simulink model "eTractor_KRAKER_etrailer_v2_2"  (R2023a)
settings: Solver=VariableStepAuto  StartTime=0.0  StopTime=tmax  FixedStep=dt  RelTol=1e-4  EnableMultiTasking=on
PreLoadFcn:
  | init_vehicle
  | init_ETruck
  | init_SIMULATION_runfile
StartFcn:
  | tic
StopFcn:
  | toc
  | sim_stop_function
values from neighbouring files (symbols this model uses):
  Arms = [100 200 300 400 500 600]    [init_BURGERS.m]    (also in init_KRAKER.m)
  brake_input = [0   tmax ... (first row only)    [init_vehicle.m]    (also in run_Circle.m = [0  tmax; run_Coastdown.m = [0  2  tmax; run_DoubleLaneChangeDriver.m = [0   2  tmax; run_MaxAcc.m = [0  2  tmax)
  chassis_length = 13.82    [init_BURGERS.m]    (also in init_KRAKER.m = 10.36)
  energyCapacity = 116.89    [init_BURGERS.m]    (also in init_KRAKER.m)
  etrailer_ON = 1    [init_SIMULATION_runfile.m]
  ETruck_energyCapacity = 650    [init_ETruck.m]
  ETruck_G_motor = 17.5    [init_ETruck.m]
  ETruck_initialSOC = 0.95    [init_ETruck.m]
  ETruck_MaxTrqOut = 2250    [init_ETruck.m]
  ETruck_Std_Regen_Trq = 300    [init_ETruck.m]
  ETruck_Voc = 750    [init_ETruck.m]
  front_overhang = 1.620    (= 1.62)    [init_BURGERS.m]    (also in init_KRAKER.m = 1.305)
  G_diff = 1    [init_BURGERS.m]    (also in init_KRAKER.m = 6)
  initialSOC = 0.95    [init_BURGERS.m]    (also in init_KRAKER.m = 0.65)
  InputSwitch = 2    [init_SIMULATION_runfile.m]
  inverter_thermal_res = 0.017    [init_BURGERS.m]    (also in init_KRAKER.m)
  L_0f = 3.8    [init_vehicle.m]
  LD = 1    [init_vehicle.m]
  mass = mass_trailer    (= 11000)    [init_BURGERS.m]    (also in init_KRAKER.m = 7350; run_Statics_MF_MAT.m = (Fz_front_axle1+Fz_rear_axle1+       Fz_trailer1_axle1+Fz_tr; run_Statics_MF_TNO.m = (Fz_front_axle1+Fz_rear_axle1+       Fz_trailer1_axle1+Fz_tr)
  massload = 23000    [init_SIMULATION_runfile.m]
  MaxTrqOut = 525    [init_BURGERS.m]    (also in init_KRAKER.m = 950)
  outside_temp = 25    [init_BURGERS.m]    (also in init_KRAKER.m)
  pose_t0 = [0 0 0 0]    [init_vehicle.m]    (also in run_Circle.m; run_Coastdown.m; run_DoubleLaneChangeDriver.m; run_MaxAcc.m)
  Power_dissipation = [261 384 513 642; 552 783 1020 1260; 894 1233 1584 1956; 1300 1750 2200 2740; 1740 2300 2900 3550; 2250 2900 3650 4500]    [init_BURGERS.m]    (also in init_KRAKER.m)
  sp_t = 0.01    [init_vehicle.m]
  Std_Regen_Trq = 300    [init_BURGERS.m]    (also in init_KRAKER.m)
  steer_input = [0  tmax ... (first row only)    [init_vehicle.m]    (also in run_Circle.m = [0  2   10     13       tmax; run_Coastdown.m = [0 tmax; run_DoubleLaneChangeDriver.m = [0 tmax; run_MaxAcc.m = [0 tmax)
  steer_ratio = 20    [init_vehicle.m]
  steer_sens = 1    [init_vehicle.m]
  throttle_input = [0         tmax ... (first row only)    [init_vehicle.m]    (also in run_Circle.m; run_Coastdown.m = [0        10         10.0001 tmax; run_DoubleLaneChangeDriver.m = [0        tmax; run_MaxAcc.m = [0        tmax)
  tire_param_drive = simscape.multibody.tirread('DRIVE_315_70R22.5_9b_MF62.tir')    [init_vehicle.m]
  tire_param_steer = simscape.multibody.tirread('STEER_315_70R22.5_9b_MF62.tir')    [init_vehicle.m]
  tire_param_trailer = simscape.multibody.tirread('TRAILER_385_65R22.5_9b0_MF62.tir')    [init_vehicle.m]
  tire_width = 0.318    [init_vehicle.m]
  trailer_ID = 1    [init_SIMULATION_runfile.m]
  v_0 = 1    [init_vehicle.m]
  Vdc = [200 400 600 800]    [init_BURGERS.m]    (also in init_KRAKER.m)
  Voc = 675    [init_BURGERS.m]    (also in init_KRAKER.m)
  Vx = 0    [init_vehicle.m]    (also in run_Circle.m = Vx_kmh/3.6; run_Coastdown.m = Vx_kmh/3.6; run_DoubleLaneChangeDriver.m = Vx_kmh/3.6; run_MaxAcc.m)
  Vx_input = [0  tmax ... (first row only)    [init_vehicle.m]    (also in run_Circle.m; run_Coastdown.m = [0 tmax; run_DoubleLaneChangeDriver.m = [0 tmax; run_MaxAcc.m = [0 tmax)
  wheelbase = 8.115    [init_BURGERS.m]    (also in init_KRAKER.m = 5.584)
undefined symbols (not defined in the file or in its folder): end_val, final_x, final_y, Floor, steer_path, X, Y, Z
libraries: sm_lib x367, nesl_utility x289, fl_lib x29, sdl_lib x4, batteryecm_lib x2, ee_lib x2, BatteryEstimators x2, robotalgslib x1, simulink_extras x1, CommercialVehicleLibrary2G x1
(part 9 of 14)

== system eTractor_KRAKER_etrailer_v2_2/Tractor_semitrailer /e-Tractor/World ==
  note: Road Vizualisation
  " pos_initial" : sm_lib/Frames and Transforms/Rigid Transform  TranslationMethod=Cartesian  TranslationStandardOffset=0  TranslationStandardOffsetUnits=m  TranslationStandardAxis=+Z  TranslationCartesianOffset=[Xt0 Yt0 0]  TranslationCartesianOffsetUnits=m  TranslationROffset=0  TranslationROffsetUnits=m  TranslationZOffset=0  TranslationZOffsetUnits=m  TranslationThetaOffset=0  TranslationThetaOffsetUnits=deg  RotationMethod=StandardAxis  RotationAngleUnits=deg  RotationStandardAxis=+Z  RotationAngle=Psit0  RotationArbitraryAxis=[0 0 1]  FollAlignAxisA=+X  BaseAlignAxisA=+Y  FollAlignAxisB=+Y  BaseAlignAxisB=+Z  RotationSequenceAxes=FollowerAxes  RotationSequence=XYX  RotationSequenceAngles=[0 0 0]  RotationSequenceAnglesUnits=deg  RotationMatrix=[1 0 0; 0 1 0; 0 0 1]  Quaternion=[1 0 0 0]
  6-DOF Joint : sm_lib/Joints/6-DOF Joint  JointMode=Normal  SenseConstraintForce=off  SenseConstraintForceX=off  SenseConstraintForceY=off  SenseConstraintForceZ=off  SenseConstraintTorque=off  SenseConstraintTorqueX=off  SenseConstraintTorqueY=off  SenseConstraintTorqueZ=off  SenseTotalForce=off  SenseTotalForceX=off  SenseTotalForceY=off  SenseTotalForceZ=off  SenseTotalTorque=off  SenseTotalTorqueX=off  SenseTotalTorqueY=off  SenseTotalTorqueZ=off  CompositeWrenchDir=BaseOnFollower  CompositeWrenchFrame=BaseFrame  PxEquilibriumPosition=0  PxEquilibriumPositionUnits=m  PxSpringStiffness=0  PxSpringStiffnessUnits=N/m  PxDampingCoefficient=0  PxDampingCoefficientUnits=N/(m/s)  PxTorqueActuationMode=NoTorque  PxMotionActuationMode=ComputedMotion  PxSensePosition=on  PxSenseVelocity=off  PxSenseAcceleration=off  PxSenseTorqueForce=off  PxSenseLowerLimitTorqueForce=off  PxSenseUpperLimitTorqueForce=off  PxLowerLimitSpecify=off  PxLowerLimitBound=-1  PxLowerLimitBoundUnits=m  PxLowerLimitStiffness=1e6  PxLowerLimitStiffnessUnits=N/m  PxLowerLimitDamping=1e3  PxLowerLimitDampingUnits=N/(m/s)  PxLowerLimitTransitionRegionWidth=1e-4  PxLowerLimitTransitionRegionWidthUnits=m  PxUpperLimitSpecify=off  PxUpperLimitBound=1  PxUpperLimitBoundUnits=m  PxUpperLimitStiffness=1e6  PxUpperLimitStiffnessUnits=N/m  PxUpperLimitDamping=1e3  PxUpperLimitDampingUnits=N/(m/s)  PxUpperLimitTransitionRegionWidth=1e-4  PxUpperLimitTransitionRegionWidthUnits=m  PxPositionTargetSpecify=off  PxPositionTargetPriority=High  PxPositionTargetValue=0  PxPositionTargetValueUnits=m  PxVelocityTargetSpecify=off  PxVelocityTargetPriority=High  PxVelocityTargetValue=Vx  PxVelocityTargetValueUnits=m/s  PyEquilibriumPosition=0  PyEquilibriumPositionUnits=m  PySpringStiffness=0  PySpringStiffnessUnits=N/m  PyDampingCoefficient=0  PyDampingCoefficientUnits=N/(m/s)  PyTorqueActuationMode=NoTorque  PyMotionActuationMode=ComputedMotion  PySensePosition=on  PySenseVelocity=off  PySenseAcceleration=off  PySenseTorqueForce=off  PySenseLowerLimitTorqueForce=off  PySenseUpperLimitTorqueForce=off  PyLowerLimitSpecify=off  PyLowerLimitBound=-1  PyLowerLimitBoundUnits=m  PyLowerLimitStiffness=1e6  PyLowerLimitStiffnessUnits=N/m  PyLowerLimitDamping=1e3  PyLowerLimitDampingUnits=N/(m/s)  PyLowerLimitTransitionRegionWidth=1e-4  PyLowerLimitTransitionRegionWidthUnits=m  PyUpperLimitSpecify=off  PyUpperLimitBound=1  PyUpperLimitBoundUnits=m  PyUpperLimitStiffness=1e6  PyUpperLimitStiffnessUnits=N/m  PyUpperLimitDamping=1e3  PyUpperLimitDampingUnits=N/(m/s)  PyUpperLimitTransitionRegionWidth=1e-4  PyUpperLimitTransitionRegionWidthUnits=m  PyPositionTargetSpecify=off  PyPositionTargetPriority=High  PyPositionTargetValue=0  PyPositionTargetValueUnits=m  PyVelocityTargetSpecify=off  PyVelocityTargetPriority=High  PyVelocityTargetValue=0  PyVelocityTargetValueUnits=m/s  PzEquilibriumPosition=0  PzEquilibriumPositionUnits=m  PzSpringStiffness=0  PzSpringStiffnessUnits=N/m  PzDampingCoefficient=0  PzDampingCoefficientUnits=N/(m/s)  PzTorqueActuationMode=NoTorque  PzMotionActuationMode=ComputedMotion  PzSensePosition=on  PzSenseVelocity=off  PzSenseAcceleration=off  PzSenseTorqueForce=off  PzSenseLowerLimitTorqueForce=off  PzSenseUpperLimitTorqueForce=off  PzLowerLimitSpecify=off  PzLowerLimitBound=-1  PzLowerLimitBoundUnits=m  PzLowerLimitStiffness=1e6  PzLowerLimitStiffnessUnits=N/m  PzLowerLimitDamping=1e3  PzLowerLimitDampingUnits=N/(m/s)  PzLowerLimitTransitionRegionWidth=1e-4  PzLowerLimitTransitionRegionWidthUnits=m  PzUpperLimitSpecify=off  PzUpperLimitBound=1  PzUpperLimitBoundUnits=m  PzUpperLimitStiffness=1e6  PzUpperLimitStiffnessUnits=N/m  PzUpperLimitDamping=1e3  PzUpperLimitDampingUnits=N/(m/s)  PzUpperLimitTransitionRegionWidth=1e-4  PzUpperLimitTransitionRegionWidthUnits=m  PzPositionTargetSpecify=off  PzPositionTargetPriority=High  PzPositionTargetValue=0  PzPositionTargetValueUnits=m  PzVelocityTargetSpecify=off  PzVelocityTargetPriority=High  PzVelocityTargetValue=0  PzVelocityTargetValueUnits=m/s  SphEqPosRotationMethod=None  SphEqPosRotationAngleUnits=deg  SphEqPosRotationStandardAxis=+Z  SphEqPosRotationAngle=0.0  SphEqPosRotationArbitraryAxis=[0 0 1]  SphEqPosFollAlignAxisA=+X  SphEqPosBaseAlignAxisA=+Y  SphEqPosFollAlignAxisB=+Y  SphEqPosBaseAlignAxisB=+Z  SphEqPosRotationSequenceAxes=FollowerAxes  SphEqPosRotationSequence=XYX  SphEqPosRotationSequenceAngles=[0 0 0]  SphEqPosRotationSequenceAnglesUnits=deg  SphEqPosRotationMatrix=[1 0 0; 0 1 0; 0 0 1]  SphEqPosQuaternion=[1 0 0 0]  SphSpringStiffness=0  SphSpringStiffnessUnits=N*m/deg  SphDampingCoefficient=0  SphDampingCoefficientUnits=N*m/(deg/s)  SphActuateTorqueX=off  SphActuateTorqueY=off  SphActuateTorqueZ=off  SphActuateTorque=off  SphTorqueActuationMode=NoTorque  SphMotionActuationMode=ComputedMotion  SphActuationFrame=BaseFrame  SphSensePosition=off  SphSenseVelocityX=off  SphSenseVelocityY=off  SphSenseVelocityZ=off  SphSenseVelocity=off  SphSenseAccelerationX=off  SphSenseAccelerationY=off  SphSenseAccelerationZ=off  SphSenseAcceleration=off  SphSenseTorqueX=off  SphSenseTorqueY=off  SphSenseTorqueZ=off  SphSenseTorqueForce=off  SphSenseLowerLimitTorqueMag=off  SphSenseUpperLimitTorqueMag=off  SphSensingFrame=BaseFrame  SphLowerLimitSpecify=off  SphLowerLimitBound=15  SphLowerLimitBoundUnits=deg  SphLowerLimitStiffness=1e4  SphLowerLimitStiffnessUnits=N*m/deg  SphLowerLimitDamping=10  SphLowerLimitDampingUnits=N*m/(deg/s)  SphLowerLimitTransitionRegionWidth=0.1  SphLowerLimitTransitionRegionWidthUnits=deg  SphUpperLimitSpecify=off  SphUpperLimitBound=45  SphUpperLimitBoundUnits=deg  SphUpperLimitStiffness=1e4  SphUpperLimitStiffnessUnits=N*m/deg  SphUpperLimitDamping=10  SphUpperLimitDampingUnits=N*m/(deg/s)  SphUpperLimitTransitionRegionWidth=0.1  SphUpperLimitTransitionRegionWidthUnits=deg  SphPositionTargetRotationMethod=None  SphPositionTargetRotationAngleUnits=deg  SphPositionTargetRotationStandardAxis=+Z  SphPositionTargetRotationAngle=0.0  SphPositionTargetRotationArbitraryAxis=[0 0 1]  SphPositionTargetFollAlignAxisA=+X  SphPositionTargetBaseAlignAxisA=+Y  SphPositionTargetFollAlignAxisB=+Y  SphPositionTargetBaseAlignAxisB=+Z  SphPositionTargetRotationSequenceAxes=FollowerAxes  SphPositionTargetRotationSequence=XYX  SphPositionTargetRotationSequenceAngles=[0 0 0]  SphPositionTargetRotationSequenceAnglesUnits=deg  SphPositionTargetRotationMatrix=[1 0 0; 0 1 0; 0 0 1]  SphPositionTargetQuaternion=[1 0 0 0]  SphPositionTargetSpecify=off  SphPositionTargetPriority=High  SphVelocityTargetValue=[0 0 0]  SphVelocityTargetValueUnits=deg/s  SphVelocityTargetSpecify=off  SphVelocityTargetPriority=High  SphVelocityTargetInFollowerFrame=on
  Bus Creator1 : BusCreator  Inputs=6
  Constant1 : Constant  Commented=on  Value=5000
  Floor : sm_lib/Body Elements/Brick Solid  GraphicAmbientColor=[0.15 0.15 0.15 1.0]  BasedOnType=Density  BrickDimensions=[Floor.l , Floor.w , Floor.h]  BrickDimensionsUnits=m  CenterOfMass=[0 0 0]  CenterOfMassUnits=m  GraphicDiffuseColor=[0.6 0.6 0.6]  Density=1000  DensityUnits=kg/(m^3)  DoExposeReferenceFrame=on  GraphicEmissiveColor=[0.0 0.0 0.0 1.0]  ExportEntireGeometry=off  SerializedFrames=<Frames/>  MarkerShape=Sphere  MarkerSize=10  GraphicType=FromGeometry  InertiaType=CalculateFromGeometry  Mass=1  MassUnits=kg  MomentsOfInertia=[1 1 1]  MomentsOfInertiaUnits=kg*m^2  GraphicOpacity=1.0  ProductsOfInertia=[0 0 0]  ProductsOfInertiaUnits=kg*m^2  GraphicShininess=75  GraphicSpecularColor=[0.5 0.5 0.5 1.0]  GraphicVisPropType=AdvancedVisualProperties
  Grid XLines : sm_lib/Body Elements/Extruded Solid  GraphicAmbientColor=[0.15 0.15 0.15 1.0]  BasedOnType=Density  CenterOfMass=[0 0 0]  CenterOfMassUnits=m  GraphicDiffuseColor=Grid.clr  ExportConvexHullGeometry=off  ExtrusionCrossSection=Grid.extr_data  ExtrusionCrossSectionUnits=m  Density=1000  DensityUnits=kg/m^3  DoExposeReferenceFrame=on  GraphicEmissiveColor=[0.0 0.0 0.0 1.0]  ExportEntireGeometry=off  ExtrusionLength=Floor.h*1.005  ExtrusionLengthUnits=m  ExtrusionType=General  SerializedFrames=<Frames/>  MarkerShape=Sphere  MarkerSize=10  GraphicType=FromGeometry  InertiaType=PointMass  Mass=1  MassUnits=kg  MomentsOfInertia=[1 1 1]  MomentsOfInertiaUnits=kg*m^2  PolygonNumSides=3  GraphicOpacity=1.0  PolygonOuterRadius=1  PolygonOuterRadiusUnits=m  ProductsOfInertia=[1 1 1]  ProductsOfInertiaUnits=kg*m^2  GraphicShininess=75  GraphicSpecularColor=[0.5 0.5 0.5 1.0]  GraphicVisPropType=SimpleVisualProperties
  Grid YLines : sm_lib/Body Elements/Extruded Solid  GraphicAmbientColor=[0.15 0.15 0.15 1.0]  BasedOnType=Density  CenterOfMass=[0 0 0]  CenterOfMassUnits=m  GraphicDiffuseColor=Grid.clr  ExportConvexHullGeometry=off  ExtrusionCrossSection=Grid.extr_data  ExtrusionCrossSectionUnits=m  Density=1000  DensityUnits=kg/m^3  DoExposeReferenceFrame=on  GraphicEmissiveColor=[0.0 0.0 0.0 1.0]  ExportEntireGeometry=off  ExtrusionLength=Floor.h*1.005  ExtrusionLengthUnits=m  ExtrusionType=General  SerializedFrames=<Frames/>  MarkerShape=Sphere  MarkerSize=10  GraphicType=FromGeometry  InertiaType=PointMass  Mass=1  MassUnits=kg  MomentsOfInertia=[1 1 1]  MomentsOfInertiaUnits=kg*m^2  PolygonNumSides=3  GraphicOpacity=1.0  PolygonOuterRadius=1  PolygonOuterRadiusUnits=m  ProductsOfInertia=[1 1 1]  ProductsOfInertiaUnits=kg*m^2  GraphicShininess=75  GraphicSpecularColor=[0.5 0.5 0.5 1.0]  GraphicVisPropType=SimpleVisualProperties
  Infinite Plane : sm_lib/Curves and Surfaces/Infinite Plane  GraphicType=Rectangle  GraphicPlaneWidth=1  GraphicPlaneWidthUnits=m  GraphicPlaneHeight=1  GraphicPlaneHeightUnits=m  GraphicVisPropType=SimpleVisualProperties  GraphicDiffuseColor=[0.5 0.5 0.5]  GraphicOpacity=0.25  GraphicSpecularColor=[0.5 0.5 0.5 1.0]  GraphicAmbientColor=[0.15 0.15 0.15 1.0]  GraphicEmissiveColor=[0.0 0.0 0.0 1.0]  GraphicShininess=75
  Mechanism Configuration : sm_lib/Utilities/Mechanism Configuration  UniformGravity=Constant  GravityVector=[0 0 -9.81]  GravityVectorUnits=m/s^2  LinearizationDelta=0.001  JointModeTransitionNonlinearIterations=2
  PS-Simulink Converter : nesl_utility/PS-Simulink Converter  PhysicalDomain=network_engine_domain  SubClassName=ps_output  LeftPortType=input  RightPortType=output  PseudoPeriodic=off  Frequencies=[]  VectorFormat=1-D array  Unit=1  AffineConversion=off
  PS-Simulink Converter1 : nesl_utility/PS-Simulink Converter  PhysicalDomain=network_engine_domain  SubClassName=ps_output  LeftPortType=input  RightPortType=output  PseudoPeriodic=off  Frequencies=[]  VectorFormat=1-D array  Unit=m  AffineConversion=off
  PS-Simulink Converter2 : nesl_utility/PS-Simulink Converter  PhysicalDomain=network_engine_domain  SubClassName=ps_output  LeftPortType=input  RightPortType=output  PseudoPeriodic=off  Frequencies=[]  VectorFormat=1-D array  Unit=m  AffineConversion=off
  PS-Simulink Converter3 : nesl_utility/PS-Simulink Converter  PhysicalDomain=network_engine_domain  SubClassName=ps_output  LeftPortType=input  RightPortType=output  PseudoPeriodic=off  Frequencies=[]  VectorFormat=1-D array  Unit=m  AffineConversion=off
  "Road Grid Offset " : sm_lib/Frames and Transforms/Rigid Transform  TranslationMethod=Cartesian  TranslationStandardOffset=0  TranslationStandardOffsetUnits=m  TranslationStandardAxis=+Z  TranslationCartesianOffset=[0 0 -0.5*Floor.h]  TranslationCartesianOffsetUnits=m  TranslationROffset=0  TranslationROffsetUnits=m  TranslationZOffset=0  TranslationZOffsetUnits=m  TranslationThetaOffset=0  TranslationThetaOffsetUnits=deg  RotationMethod=None  RotationAngleUnits=deg  RotationStandardAxis=+Z  RotationAngle=45  RotationArbitraryAxis=[0 0 1]  FollAlignAxisA=+X  BaseAlignAxisA=+Y  FollAlignAxisB=+Y  BaseAlignAxisB=+Z  RotationSequenceAxes=FollowerAxes  RotationSequence=XYX  RotationSequenceAngles=[0 0 0]  RotationSequenceAnglesUnits=deg  RotationMatrix=[1 0 0; 0 1 0; 0 0 1]  Quaternion=[1 0 0 0]
  Simulink-PS Converter : nesl_utility/Simulink-PS Converter  Commented=on  PhysicalDomain=network_engine_domain  SubClassName=ps_input  LeftPortType=input  RightPortType=output  PseudoPeriodic=off  Frequencies=[]  NoiseDistribution=none  NoiseParameters=[]  Unit=N  AffineConversion=off  FilteringAndDerivatives=provide  SimscapeFilterOrder=1  InputFilterTimeConstant=0.001  UdotUserProvided=0
  Solver Configuration : nesl_utility/Solver Configuration  PhysicalDomain=network_engine_domain  SubClassName=solver  LeftPortType=input  RightPortType=generic  Tones=[]  Harmonics=[]  SimulateNoise=off  Profile=off  UseLocalSampling=off  EnableSwitchedLinearOptims=on  FrequencyDomain=off  UseCCode=off  RelTol=0.001  AbsTol=1e-06  MinStep=1e-09  ToWorkspace=off  RevertToSquareIcSolve=off  NumHomotopyIterations=100  PhasorMode=off  PhasorModeNumHarmonics=1  ConsistencySolver=NEWTON_FTOL  IndexReductionMethod=DerivativeReplacement  DoDC=off  ResidualTolerance=1e-09  ConsistencyTolSource=GLOBAL  ConsistencyAbsTol=0.001  ConsistencyRelTol=0.001  ConsistencyTolFactor=0.001  UseLocalSolver=off  LocalSolverChoice=NE_BACKWARD_EULER_ADVANCER  ResolveIndetEquations=on  FunctionEvalNumThread=1  LocalSolverSampleTime=0.001  DoFixedCost=off  MaxNonlinIter=3  MaxModeIter=2  ComputeImpulses=off  ImpulseIterations=2  LinearAlgebra=Sparse  LinearAlgebraNumThread=0  EquationFormulation=NE_TIME_EF  DelaysMemoryBudget=1024  AutomaticFiltering=on  FilteringTimeConstant=0.001  PartitionStorageMethod=AS_NEEDED  PartitionMemoryBudget=1024  PartitionMethod=ROBUST
  Step : Step  Commented=on  Time=10  After=25000  SampleTime=0
  Subsystem : Subsystem
      mask Display: disp('Yaw, Pitch & Roll');
  Transform Sensor : sm_lib/Frames and Transforms/Transform Sensor  MeasurementFrame=World  RotationSequence=XYX  SenseAngle=off  SenseAxis=off  SenseQ=off  SenseR=on  SenseRotationSequence=off  SenseOmegaX=off  SenseOmegaY=off  SenseOmegaZ=off  SenseQDot=off  SenseRDot=off  SenseRotationSequenceDot=off  SenseAlphaX=off  SenseAlphaY=off  SenseAlphaZ=off  SenseQDDot=off  SenseRDDot=off  SenseX=off  SenseY=off  SenseZ=off  SenseRad=off  SenseAzim=off  SenseDist=off  SenseInc=off  SenseXDot=off  SenseYDot=off  SenseZDot=off  SenseRadDot=off  SenseAzimDot=off  SenseDistDot=off  SenseIncDot=off  SenseXDDot=off  SenseYDDot=off  SenseZDDot=off  SenseRadDDot=off  SenseAzimDDot=off  SenseDistDDot=off  SenseIncDDot=off
  "Transform XLines " : sm_lib/Frames and Transforms/Rigid Transform  TranslationMethod=Cartesian  TranslationStandardOffset=0  TranslationStandardOffsetUnits=m  TranslationStandardAxis=+Z  TranslationCartesianOffset=[0 0 0]  TranslationCartesianOffsetUnits=m  TranslationROffset=0  TranslationROffsetUnits=m  TranslationZOffset=0  TranslationZOffsetUnits=m  TranslationThetaOffset=0  TranslationThetaOffsetUnits=deg  RotationMethod=StandardAxis  RotationAngleUnits=deg  RotationStandardAxis=+Z  RotationAngle=90  RotationArbitraryAxis=[0 0 1]  FollAlignAxisA=+X  BaseAlignAxisA=+Y  FollAlignAxisB=+Y  BaseAlignAxisB=+Z  RotationSequenceAxes=FollowerAxes  RotationSequence=XYX  RotationSequenceAngles=[0 0 0]  RotationSequenceAnglesUnits=deg  RotationMatrix=[1 0 0; 0 1 0; 0 0 1]  Quaternion=[1 0 0 0]
  Transport Delay (for initial settling period)1 : TransportDelay  Commented=on  DelayTime=5
  World Frame : sm_lib/Frames and Transforms/World Frame
  pos_chas_front : sm_lib/Frames and Transforms/Rigid Transform  TranslationMethod=Cartesian  TranslationStandardOffset=0  TranslationStandardOffsetUnits=m  TranslationStandardAxis=+Z  TranslationCartesianOffset=[-xcg_front 0 0.9]  TranslationCartesianOffsetUnits=m  TranslationROffset=0  TranslationROffsetUnits=m  TranslationZOffset=0  TranslationZOffsetUnits=m  TranslationThetaOffset=0  TranslationThetaOffsetUnits=deg  RotationMethod=None  RotationAngleUnits=deg  RotationStandardAxis=+Z  RotationAngle=0.0  RotationArbitraryAxis=[0 0 1]  FollAlignAxisA=+X  BaseAlignAxisA=+Y  FollAlignAxisB=+Y  BaseAlignAxisB=+Z  RotationSequenceAxes=FollowerAxes  RotationSequence=XYX  RotationSequenceAngles=[0 0 0]  RotationSequenceAnglesUnits=deg  RotationMatrix=[1 0 0; 0 1 0; 0 0 1]  Quaternion=[1 0 0 0]
  Road : PMIOPort  Side=Left
  Measurements : PMIOPort  Port=2  Side=Left
  Chassis : PMIOPort  Port=3  Side=Right
  signals : Outport
  wires:
  PS-Simulink Converter/1 -> Subsystem/1(In1)
  Subsystem/2(pitch) -> Bus Creator1/5
  Subsystem/3(roll) -> Bus Creator1/6
  Bus Creator1/1 -> signals/1
  PS-Simulink Converter1/1 -> Bus Creator1/1  "X"
  PS-Simulink Converter2/1 -> Bus Creator1/2  "Y"
  PS-Simulink Converter3/1 -> Bus Creator1/3  "Z"
  Subsystem/1(yaw) -> Bus Creator1/4
  Step/1 -> Simulink-PS Converter/1
  Constant1/1 -> Transport Delay (for initial settling period)1/1
  connections:
  Grid XLines/RConn1 -- "Transform XLines "/RConn1
  pos_chas_front/RConn1 -- Measurements/RConn1 -- 6-DOF Joint/LConn1
  Solver Configuration/RConn1 -- Infinite Plane/LConn1 -- Transform Sensor/LConn1 -- " pos_initial"/LConn1 -- "Road Grid Offset "/LConn1 -- World Frame/RConn1 -- Mechanism Configuration/RConn1
  "Road Grid Offset "/RConn1 -- Floor/RConn1 -- "Transform XLines "/LConn1 -- Grid YLines/RConn1
  " pos_initial"/RConn1 -- pos_chas_front/LConn1
  6-DOF Joint/RConn1 -- Transform Sensor/RConn1 -- Chassis/RConn1
  PS-Simulink Converter/LConn1 -- Transform Sensor/RConn2
  PS-Simulink Converter3/LConn1 -- 6-DOF Joint/RConn4
  PS-Simulink Converter2/LConn1 -- 6-DOF Joint/RConn3
  PS-Simulink Converter1/LConn1 -- 6-DOF Joint/RConn2
  Road/RConn1 -- Infinite Plane/RConn1

== system eTractor_KRAKER_etrailer_v2_2/Tractor_semitrailer /Driver/Control/Pure persuit controller ==
  Pose : Inport
  Waypoints : Inport  Port=2
  Atan : Trigonometry  Operator=atan
  Constant : Constant  Value=L_0f
  Constant1 : Constant  Value=LD
  Constant2 : Constant  Value=v_0
  Constant3 : Constant  Value=2
  Divide : Product  Inputs=*/
  Product : Product  Inputs=3
  Product1 : Product
  Pure Pursuit : robotalgslib/Pure Pursuit  DesiredLinearVelocity=1  MaxAngularVelocity=0.1  LookaheadDistance=LD  TargetDirPort=on  SimulateUsing=Code generation
  Sign : Signum
  Sin : Trigonometry
  Terminator : Terminator
  Terminator1 : Terminator
  To Workspace : ToWorkspace  VariableName=targetdir  SampleTime=-1
  distance to react1 : Saturate  UpperLimit=1  LowerLimit=-1
  Delta : Outport
  wires:
  Pose/1 -> Pure Pursuit/1
  Waypoints/1 -> Pure Pursuit/2
  Sin/1 -> Product/3
  Atan/1 -> distance to react1/1
  Constant/1 -> Product/2
  Constant1/1 -> Divide/2
  Constant3/1 -> Product/1
  distance to react1/1 -> Product1/2
  Sign/1 -> Product1/1
  Pure Pursuit/3 -> Sin/1, To Workspace/1
  Pure Pursuit/2 -> Terminator1/1
  Constant2/1 -> Sign/1
  Divide/1 -> Atan/1
  Product/1 -> Divide/1
  Pure Pursuit/1 -> Terminator/1
  Product1/1 -> Delta/1

== system eTractor_KRAKER_etrailer_v2_2/Tractor_semitrailer /Driver/Control/Simulation end module ==
  x : Inport
  y : Inport  Port=2
  Cast To Boolean : DataTypeConversion  OutDataTypeStr=boolean  SaturateOnIntegerOverflow=off  RndMeth=Floor
  Constant : Constant  Commented=on  Value=end_val
  Constant1 : Constant  Commented=on  Value=end_val
  Constant2 : Constant  Commented=on  Value=v_0
  Constant3 : Constant  Value=final_x
  Constant4 : Constant  Value=final_y
  Constant5 : Constant  Value=0.5
  GreaterThan : RelationalOperator  Commented=on  Operator=<  OutDataTypeStr=boolean  RndMeth=Simplest  InputSameDT=off
  GreaterThan1 : RelationalOperator  Commented=on  Operator=<  OutDataTypeStr=boolean  RndMeth=Simplest  InputSameDT=off
  Less Than : RelationalOperator  Operator=<  OutDataTypeStr=boolean  RndMeth=Simplest  InputSameDT=off
  Scope : Scope
  Sign : Signum  Commented=on
  Sqrt : Sqrt
  Square : Math  Operator=square
  Square1 : Math  Operator=square
  Stop Simulation : Stop  Commented=on
  Stop Simulation1 : Stop
  Sum : Sum
  Sum1 : Sum  Inputs=+-
  Sum2 : Sum  Inputs=+-
  Switch : Switch  Commented=on  Criteria=u2 > Threshold  SaturateOnIntegerOverflow=off  InputSameDT=off
  wires:
  Constant5/1 -> Less Than/2
  Sqrt/1 -> Less Than/1, Scope/1
  Constant4/1 -> Sum2/2
  Sum2/1 -> Square1/1
  Sum1/1 -> Square/1
  Constant3/1 -> Sum1/2
  Sum/1 -> Sqrt/1
  Square1/1 -> Sum/2
  Square/1 -> Sum/1
  Constant/1 -> GreaterThan/2
  x/1 -> Sum1/1
  y/1 -> Sum2/1
  Constant1/1 -> GreaterThan1/2
  Switch/1 -> Stop Simulation/1
  Sign/1 -> Switch/2
  GreaterThan/1 -> Switch/1
  GreaterThan1/1 -> Switch/3
  Constant2/1 -> Sign/1
  Less Than/1 -> Cast To Boolean/1
  Cast To Boolean/1 -> Stop Simulation1/1

== system eTractor_KRAKER_etrailer_v2_2/Tractor_semitrailer /KRAKER e-trailer/Electric Powertrain/Inverter_losses ==
  V_bat : Inport
  Current : Inport  Port=2
  Abs : Abs  SaturateOnIntegerOverflow=off
  Constant : Constant  Value=inverter_thermal_res
  Integrator : Integrator  InitialCondition=outside_temp
  Inverter power dissipation : Lookup_n-D  BreakpointsForDimension1=Arms  BreakpointsForDimension2=Vdc  Table=Power_dissipation  InternalRulePriority=Speed  RndMeth=Simplest
      settings: InputPortMap=u0,u1
  Product : Product
  To Workspace1 : ToWorkspace  VariableName=p_inverter_deltatemp  SampleTime=sp_t
  To Workspace6 : ToWorkspace  VariableName=p_inverter_powdiss  SampleTime=sp_t
  Inverter_temp_[C] : Outport
  wires:
  V_bat/1 -> Inverter power dissipation/2
  Current/1 -> Abs/1
  Abs/1 -> Inverter power dissipation/1
  Inverter power dissipation/1 -> Product/1, To Workspace6/1  "pow_diss_[W]"
  Integrator/1 -> Inverter_temp_[C]/1
  Product/1 -> Integrator/1, To Workspace1/1
  Constant/1 -> Product/2

== system eTractor_KRAKER_etrailer_v2_2/Tractor_semitrailer /KRAKER e-trailer/Electric Powertrain/SOC calculation ==
  Voc : Inport
  1/EnergyCapacity : Gain  Gain=1/(energyCapacity*Voc*3600)
  Constant1 : Constant  Value=initialSOC
  Current Sensor : fl_lib/Electrical/Electrical Sensors/Current Sensor
  Gain : Gain  Gain=-1
  Gain1 : Gain  Gain=100
  Gain2 : Gain  Gain=100
  Integrator : Integrator  InitialCondition=energyCapacity*Voc*3600*initialSOC
  PS-Simulink Converter1 : nesl_utility/PS-Simulink Converter  PhysicalDomain=network_engine_domain  SubClassName=ps_output  LeftPortType=input  RightPortType=output  PseudoPeriodic=off  Frequencies=[]  VectorFormat=1-D array  Unit=A  AffineConversion=off
  Product : Product
  SOC Estimator (Coulomb Counting) : BatteryEstimators/SOC Estimator (Coulomb Counting)  AH=energyCapacity  Ts=-1
      link override Integrator: LabelModeActiveChoice=Discrete
      settings: LibrarySourceBlock=|
      | batt_sl_lib/Estimators/SOC Estimator
      | (Coulomb Counting)
  Scope : Scope
  + : PMIOPort  Side=Left
  - : PMIOPort  Port=2  Side=Right
  SOC_Coulomb : Outport
  Current : Outport  Port=2
  SOC_calc : Outport  Port=3
  wires:
  Constant1/1 -> SOC Estimator (Coulomb Counting)/2
  SOC Estimator (Coulomb Counting)/1 -> Gain1/1  "SOC"
  Gain/1 -> Product/1, Current/1, SOC Estimator (Coulomb Counting)/1
  PS-Simulink Converter1/1 -> Gain/1
  Gain1/1 -> SOC_Coulomb/1
  Voc/1 -> Scope/1, Product/2
  Product/1 -> Integrator/1
  Integrator/1 -> 1/EnergyCapacity/1
  1/EnergyCapacity/1 -> Gain2/1
  Gain2/1 -> SOC_calc/1
  connections:
  Current Sensor/RConn2 -- -/RConn1
  PS-Simulink Converter1/LConn1 -- Current Sensor/RConn1
  Current Sensor/LConn1 -- +/RConn1

== system eTractor_KRAKER_etrailer_v2_2/Tractor_semitrailer /KRAKER e-trailer/Electric Powertrain/Speed Sensor ==
  Mechanical Rotational Reference1 : fl_lib/Mechanical/Rotational Elements/Mechanical Rotational Reference
  Motion Sensor : fl_lib/Mechanical/Mechanical Sensors/Ideal Rotational Motion Sensor  reference=foundation.enum.MeasurementReference.difference  acceleration_port=false  velocity_port=true  position_port=true  wrap_angle=simscape.enum.onoff.off  offset=0 rad
  PS Terminator : fl_lib/Physical Signals/Sinks/PS Terminator
  PS-Simulink Converter 2 : nesl_utility/PS-Simulink Converter  PhysicalDomain=network_engine_domain  SubClassName=ps_output  LeftPortType=input  RightPortType=output  PseudoPeriodic=off  Frequencies=[]  VectorFormat=1-D array  Unit=rpm  AffineConversion=off
  R : PMIOPort  Side=Left
  w : Outport
  wires:
  PS-Simulink Converter 2/1 -> w/1
  connections:
  Motion Sensor/RConn2 -- PS-Simulink Converter 2/LConn1
  Motion Sensor/RConn1 -- Mechanical Rotational Reference1/LConn1
  Motion Sensor/RConn3 -- PS Terminator/LConn1
  Motion Sensor/LConn1 -- R/RConn1

== system eTractor_KRAKER_etrailer_v2_2/Tractor_semitrailer /KRAKER e-trailer/Etrailer-Controller/Control ==
  Vx : Inport  Unit=m/s
  SpdRef : Inport  Port=2  Unit=m/s
  throttle : Inport  Port=3
  brake : Inport  Port=4
  Mb_trailer : Inport  Port=5
  SOC : Inport  Port=6
  Add : Sum
  Add1 : Sum  Inputs=+-
  Constant : Constant  Value=etrailer_ON
  Constant1 : Constant  Value=0
  Constant2 : Constant  Value=Std_Regen_Trq
  Control_Scope : Scope  NumInputPorts=4
  Gain : Gain  Gain=MaxTrqOut
  Gain1 : Gain  Gain=-MaxTrqOut
  Gain2 : Gain  Gain=G_diff
  Gain3 : Gain  Gain=-1
  Gain4 : Gain  Gain=1/G_diff
  MATLAB Function : MATLAB Function  TreatAsAtomicUnit=on
  Mux2 : Mux  Inputs=2
  Only Negative Trq : Saturate  UpperLimit=0  LowerLimit=-inf  ZeroCross=off
  Saturation : Saturate  UpperLimit=inf  LowerLimit=0
  Saturation1 : Saturate  UpperLimit=0  LowerLimit=-inf
  Saturation2 : Saturate  UpperLimit=0  LowerLimit=-inf
  Saturation3 : Saturate  UpperLimit=MaxTrqOut  LowerLimit=-MaxTrqOut
  Switch : Switch  Criteria=u2 > Threshold  SaturateOnIntegerOverflow=off  InputSameDT=off
  Mbrake : Outport
  TrqReq : Outport  Port=2  Unit=N*m  VectorParamsAs1DForOutWhenUnconnected=off
  wires:
  throttle/1 -> MATLAB Function/3(throttle), Gain/1
  brake/1 -> Gain1/1
  Gain/1 -> Saturation/1
  Gain1/1 -> Saturation1/1
  Saturation1/1 -> Add/2
  Saturation/1 -> Add/1
  Add/1 -> MATLAB Function/2(Torqreq)
  Mb_trailer/1 -> Gain3/1
  MATLAB Function/1(TrqReq) -> Saturation3/1
  Add1/1 -> Only Negative Trq/1  "brake_error"
  Only Negative Trq/1 -> [Mbrake_trailer], Mbrake/1  "Mbrake"
  SpdRef/1 -> Mux2/2  "Vx_ref"
  Vx/1 -> [Vx], Mux2/1  "Vx"
  Mux2/1 -> [speed_comp]
  SOC/1 -> Control_Scope/4
  [speed_comp] -> Control_Scope/1
  [Mbrake_trailer] -> Control_Scope/2
  [TrqReq] -> Control_Scope/3
  Gain2/1 -> Saturation2/1
  Saturation2/1 -> Add1/2
  Switch/1 -> Gain2/1, [TrqReq], TrqReq/1  "Torque_Req"
  Constant/1 -> Switch/2
  Constant1/1 -> Switch/3
  Gain3/1 -> Add1/1, Gain4/1
  Gain4/1 -> MATLAB Function/1(Mbtrailer)
  Saturation3/1 -> Switch/1
  Constant2/1 -> MATLAB Function/4(Std_Regen_Trq)
  [Vx] -> MATLAB Function/5(Vx)

== system eTractor_KRAKER_etrailer_v2_2/Tractor_semitrailer /KRAKER e-trailer/Trailer axle 1/Brake//Wheel_bearing ==
  Mdrive : Inport
  Mbrake : Inport  Port=2
  Gain : Gain  Gain=-1
  Look-Up Table : Lookup  InputValues=[-5:0.05:5]  Table=-tanh(2*[-5:0.05:5])
  Product1 : Product  InputSameDT=on  SaturateOnIntegerOverflow=on  OutDataTypeStr=Inherit: Same as first input
  Rotational joint around y axis : Subsystem
  Sum : Sum  Inputs=++|
  axle : PMIOPort  Side=Left
  wheel : PMIOPort  Port=2  Side=Right
  omega : Outport  VectorParamsAs1DForOutWhenUnconnected=off
  wires:
  Mbrake/1 -> Gain/1
  Look-Up Table/1 -> Product1/2
  Product1/1 -> Sum/2
  Mdrive/1 -> Sum/1
  Rotational joint around y axis/1(Rotational speed) -> omega/1, Look-Up Table/1
  Sum/1 -> Rotational joint around y axis/1(Torque)
  Gain/1 -> Product1/1
  connections:
  Rotational joint around y axis/LConn1 -- axle/RConn1
  wheel/RConn1 -- Rotational joint around y axis/RConn1

== system eTractor_KRAKER_etrailer_v2_2/Tractor_semitrailer /KRAKER e-trailer/Trailer axle 1/Brake//Wheel_bearing1 ==
  Mdrive : Inport
  Mbrake : Inport  Port=2
  Gain : Gain  Gain=-1
  Look-Up Table : Lookup  InputValues=[-5:0.05:5]  Table=-tanh(2*[-5:0.05:5])
  Product1 : Product  InputSameDT=on  SaturateOnIntegerOverflow=on  OutDataTypeStr=Inherit: Same as first input
  Rotational joint around y axis : Subsystem
  Sum : Sum  Inputs=++|
  axle : PMIOPort  Side=Left
  wheel : PMIOPort  Port=2  Side=Right
  omega : Outport  VectorParamsAs1DForOutWhenUnconnected=off
  wires:
  Mbrake/1 -> Gain/1
  Look-Up Table/1 -> Product1/2
  Product1/1 -> Sum/2
  Mdrive/1 -> Sum/1
  Rotational joint around y axis/1(Rotational speed) -> omega/1, Look-Up Table/1
  Sum/1 -> Rotational joint around y axis/1(Torque)
  Gain/1 -> Product1/1
  connections:
  Rotational joint around y axis/LConn1 -- axle/RConn1
  wheel/RConn1 -- Rotational joint around y axis/RConn1

== system eTractor_KRAKER_etrailer_v2_2/Tractor_semitrailer /KRAKER e-trailer/Trailer axle 1/Wheel FL ==
  Bus Creator : BusCreator  Inputs=6
  Bus Creator2 : BusCreator  Inputs=3
  Demux : Demux  Outputs=3
  Demux1 : Demux  Outputs=3
  Geometry Transform : sm_lib/Frames and Transforms/Rigid Transform  TranslationMethod=None  TranslationStandardOffset=0  TranslationStandardOffsetUnits=m  TranslationStandardAxis=+Y  TranslationCartesianOffset=[0 0 0]  TranslationCartesianOffsetUnits=m  TranslationROffset=0  TranslationROffsetUnits=m  TranslationZOffset=0  TranslationZOffsetUnits=m  TranslationThetaOffset=0  TranslationThetaOffsetUnits=deg  RotationMethod=StandardAxis  RotationAngleUnits=deg  RotationStandardAxis=+Z  RotationAngle=sideR*90  RotationArbitraryAxis=[0 0 1]  FollAlignAxisA=+X  BaseAlignAxisA=+Y  FollAlignAxisB=+Y  BaseAlignAxisB=+Z  RotationSequenceAxes=FollowerAxes  RotationSequence=XYX  RotationSequenceAngles=[0 0 0]  RotationSequenceAnglesUnits=deg  RotationMatrix=[1 0 0; 0 1 0; 0 0 1]  Quaternion=[1 0 0 0]
  Inertia : sm_lib/Body Elements/Inertia  InertiaType=Custom  Mass=wheelbody_mass  MassUnits=kg  CenterOfMass=[0 0 0]  CenterOfMassUnits=m  MomentsOfInertia=[Imat(1,1) Imat(2,2) Imat(3,3)]  MomentsOfInertiaUnits=kg*m^2  ProductsOfInertia=[0 0 0]  ProductsOfInertiaUnits=kg*m^2  GraphicType=None  MarkerShape=Inertia  MarkerSize=20  GraphicVisPropType=SimpleVisualProperties  GraphicDiffuseColor=[0.5 0.5 0.5]  GraphicSpecularColor=[0.5 0.5 0.5 1.0]  GraphicAmbientColor=[0.15 0.15 0.15 1.0]  GraphicEmissiveColor=[0.0 0.0 0.0 1.0]  GraphicShininess=75  GraphicOpacity=1.0
  MF Tire FL : sm_lib/Forces and Torques/Magic Formula Tire Force and Torque  TireSide=Left  TireParameters=tire_param  SlipMode=Combined  NumericParameters=[0.1 0.1 0.1 0.1 5.0 1e-4 1e-4 1e-7 1e-7 1e-4 1e-4 0.1 1e-4 1e-4 1e-4 1e-4 1e-4 1e-4 1e-4 1e-4 1e-4]  ScalingCoefficientLMUXMode=FromTireParameters  ScalingCoefficientLMUYMode=FromTireParameters  TireWrenchFrame=ContactFrame  SenseTireForce=on  SenseTireTorque=on  SensePneumaticTrail=off  SenseLongitudinalSlip=off  SenseSaturatedLongitudinalSlip=off  SenseSlipAngle=off  SenseSaturatedSlipAngle=off  SenseTurnSlip=off  SenseRelativeLongitudinalVelocity=off  SenseRelativeLateralVelocity=off  SenseLongitudinalSlipVelocity=off  SenseLateralSlipVelocity=off  SenseYawVelocity=off  SenseCamberAngle=off  SenseSaturatedCamberAngle=off  SenseCamberVelocity=off  SenseSpinVelocity=off  SenseFreeRadius=off  SenseLoadedRadius=off  SenseEffectiveRollingRadius=off  SenseLongitudinalFrictionCoefficient=off  SenseLateralFrictionCoefficient=off  SenseContactBaseRotation=off  SenseContactBaseTranslation=off  SenseContactFollowerRotation=off  SenseContactFollowerTranslation=off
  PS-Simulink Converter : nesl_utility/PS-Simulink Converter  PhysicalDomain=network_engine_domain  SubClassName=ps_output  LeftPortType=input  RightPortType=output  PseudoPeriodic=off  Frequencies=[]  VectorFormat=inherit  Unit=inherit  AffineConversion=off
  PS-Simulink Converter1 : nesl_utility/PS-Simulink Converter  PhysicalDomain=network_engine_domain  SubClassName=ps_output  LeftPortType=input  RightPortType=output  PseudoPeriodic=off  Frequencies=[]  VectorFormat=inherit  Unit=inherit  AffineConversion=off
  PS-Simulink Converter{2..11} (10 alike) : nesl_utility/PS-Simulink Converter  PhysicalDomain=network_engine_domain  SubClassName=ps_output  LeftPortType=input  RightPortType=output  PseudoPeriodic=off  Frequencies=[]  VectorFormat=1-D array  Unit=1  AffineConversion=off
  Reshape : Reshape
  Rigid Transform : sm_lib/Frames and Transforms/Rigid Transform  TranslationMethod=StandardAxis  TranslationStandardOffset=tire_width/2  TranslationStandardOffsetUnits=m  TranslationStandardAxis=+Z  TranslationCartesianOffset=[0 0 0]  TranslationCartesianOffsetUnits=m  TranslationROffset=0  TranslationROffsetUnits=m  TranslationZOffset=0  TranslationZOffsetUnits=m  TranslationThetaOffset=0  TranslationThetaOffsetUnits=deg  RotationMethod=None  RotationAngleUnits=deg  RotationStandardAxis=+Z  RotationAngle=0.0  RotationArbitraryAxis=[0 0 1]  FollAlignAxisA=+X  BaseAlignAxisA=+Y  FollAlignAxisB=+Y  BaseAlignAxisB=+Z  RotationSequenceAxes=FollowerAxes  RotationSequence=XYX  RotationSequenceAngles=[0 0 0]  RotationSequenceAnglesUnits=deg  RotationMatrix=[1 0 0; 0 1 0; 0 0 1]  Quaternion=[1 0 0 0]
  Rim+Tire : sm_lib/Body Elements/File Solid  ExtGeomFileName=wheel.STP  UnitType=Custom  ExtGeomFileUnits=mm  StepReaderType=HEX  ExportConvexHullGeometry=off  InertiaType=Custom  Mass=0  MassUnits=kg  CenterOfMass=[0 0 0]  CenterOfMassUnits=m  MomentsOfInertia=[0 0 0]  MomentsOfInertiaUnits=kg*m^2  ProductsOfInertia=[0 0 0]  ProductsOfInertiaUnits=kg*m^2  BasedOnType=Density  Density=1000  DensityUnits=kg/(m^3)  DoExposeReferenceFrame=on  SerializedFrames=<Frames/>  GraphicType=FromGeometry  MarkerShape=Sphere  MarkerSize=10  GraphicVisPropType=SimpleVisualProperties  GraphicDiffuseColor=[0.8 0.8 0.8]  GraphicSpecularColor=[0.5 0.5 0.5 1.0]  GraphicAmbientColor=[0.15 0.15 0.15 1.0]  GraphicEmissiveColor=[0.0 0.0 0.0 1.0]  GraphicShininess=75  GraphicOpacity=1.0
  Rotation Axis Transform : sm_lib/Frames and Transforms/Rigid Transform  TranslationMethod=None  TranslationStandardOffset=0  TranslationStandardOffsetUnits=m  TranslationStandardAxis=+Z  TranslationCartesianOffset=[0 0 0]  TranslationCartesianOffsetUnits=m  TranslationROffset=0  TranslationROffsetUnits=m  TranslationZOffset=0  TranslationZOffsetUnits=m  TranslationThetaOffset=0  TranslationThetaOffsetUnits=deg  RotationMethod=AlignedAxes  RotationAngleUnits=deg  RotationStandardAxis=-X  RotationAngle=0  RotationArbitraryAxis=[0 0 1]  FollAlignAxisA=+X  BaseAlignAxisA=+X  FollAlignAxisB=+Z  BaseAlignAxisB=+Y  RotationSequenceAxes=FollowerAxes  RotationSequence=XYX  RotationSequenceAngles=[0 0 0]  RotationSequenceAnglesUnits=deg  RotationMatrix=[1 0 0; 0 1 0; 0 0 1]  Quaternion=[1 0 0 0]
  Terminator{,1..6} (7 alike) : Terminator
  Transform Sensor-LocalBodyCS : sm_lib/Frames and Transforms/Transform Sensor  MeasurementFrame=NonRotatingFollower  RotationSequence=XYX  SenseAngle=off  SenseAxis=off  SenseQ=off  SenseR=off  SenseRotationSequence=off  SenseOmegaX=on  SenseOmegaY=on  SenseOmegaZ=on  SenseQDot=off  SenseRDot=off  SenseRotationSequenceDot=off  SenseAlphaX=off  SenseAlphaY=off  SenseAlphaZ=off  SenseQDDot=off  SenseRDDot=off  SenseX=off  SenseY=off  SenseZ=off  SenseRad=off  SenseAzim=off  SenseDist=off  SenseInc=off  SenseXDot=on  SenseYDot=on  SenseZDot=on  SenseRadDot=off  SenseAzimDot=off  SenseDistDot=off  SenseIncDot=off  SenseXDDot=off  SenseYDDot=off  SenseZDDot=off  SenseRadDDot=off  SenseAzimDDot=off  SenseDistDDot=off  SenseIncDDot=off
  Transform Sensor-WorldCS : sm_lib/Frames and Transforms/Transform Sensor  MeasurementFrame=World  RotationSequence=XYX  SenseAngle=off  SenseAxis=off  SenseQ=off  SenseR=on  SenseRotationSequence=off  SenseOmegaX=off  SenseOmegaY=off  SenseOmegaZ=off  SenseQDot=off  SenseRDot=off  SenseRotationSequenceDot=off  SenseAlphaX=off  SenseAlphaY=off  SenseAlphaZ=off  SenseQDDot=off  SenseRDDot=off  SenseX=on  SenseY=on  SenseZ=on  SenseRad=off  SenseAzim=off  SenseDist=off  SenseInc=off  SenseXDot=off  SenseYDot=off  SenseZDot=off  SenseRadDot=off  SenseAzimDot=off  SenseDistDot=off  SenseIncDot=off  SenseXDDot=off  SenseYDDot=off  SenseZDDot=off  SenseRadDDot=off  SenseAzimDDot=off  SenseDistDDot=off  SenseIncDDot=off
  World Frame : sm_lib/Frames and Transforms/World Frame
  "Wheel " : PMIOPort  Side=Left
  Ground : PMIOPort  Port=2  Side=Left
  Tire Foces : Outport
  Tire Position : Outport  Port=2
  wires:
  PS-Simulink Converter/1 -> Demux/1
  Demux/2 -> Bus Creator/2  "Lateral: Fy"
  Bus Creator/1 -> Tire Foces/1
  Demux/3 -> Bus Creator/3  "Normal: Fz"
  PS-Simulink Converter1/1 -> Demux1/1
  Demux1/2 -> Bus Creator/5  "Rolling Resistance: My"
  Demux1/3 -> Bus Creator/6  "Aligning: Mz"
  Demux1/1 -> Bus Creator/4  "Overturning: Mx"
  Demux/1 -> Bus Creator/1  "Longitudinal: Fx"
  PS-Simulink Converter6/1 -> Terminator1/1  "wx"
  PS-Simulink Converter10/1 -> Terminator5/1  "vy"
  PS-Simulink Converter8/1 -> Terminator3/1  "wz"
  PS-Simulink Converter2/1 -> Reshape/1
  PS-Simulink Converter9/1 -> Terminator4/1  "vx"
  PS-Simulink Converter5/1 -> Bus Creator2/3  "z"
  Bus Creator2/1 -> Tire Position/1
  PS-Simulink Converter7/1 -> Terminator2/1  "wy"
  Reshape/1 -> Terminator/1  "R"
  PS-Simulink Converter3/1 -> Bus Creator2/1  "x"
  PS-Simulink Converter4/1 -> Bus Creator2/2  "y"
  PS-Simulink Converter11/1 -> Terminator6/1  "vz"
  connections:
  PS-Simulink Converter1/LConn1 -- MF Tire FL/RConn3
  PS-Simulink Converter/LConn1 -- MF Tire FL/RConn2
  Ground/RConn1 -- MF Tire FL/LConn1
  Transform Sensor-LocalBodyCS/RConn1 -- Rotation Axis Transform/RConn1 -- "Wheel "/RConn1 -- MF Tire FL/RConn1 -- Rigid Transform/LConn1
  Rim+Tire/RConn1 -- Geometry Transform/RConn1
  Geometry Transform/LConn1 -- Inertia/RConn1 -- Rotation Axis Transform/LConn1
  Transform Sensor-LocalBodyCS/LConn1 -- World Frame/RConn1 -- Transform Sensor-WorldCS/LConn1
  Transform Sensor-WorldCS/RConn1 -- Rigid Transform/RConn1
  Transform Sensor-WorldCS/RConn4 -- PS-Simulink Converter4/LConn1
  Transform Sensor-LocalBodyCS/RConn7 -- PS-Simulink Converter11/LConn1
  Transform Sensor-LocalBodyCS/RConn5 -- PS-Simulink Converter9/LConn1
  Transform Sensor-WorldCS/RConn2 -- PS-Simulink Converter2/LConn1
  Transform Sensor-WorldCS/RConn5 -- PS-Simulink Converter5/LConn1
  Transform Sensor-LocalBodyCS/RConn2 -- PS-Simulink Converter6/LConn1
  Transform Sensor-WorldCS/RConn3 -- PS-Simulink Converter3/LConn1
  Transform Sensor-LocalBodyCS/RConn3 -- PS-Simulink Converter7/LConn1
  Transform Sensor-LocalBodyCS/RConn4 -- PS-Simulink Converter8/LConn1
  Transform Sensor-LocalBodyCS/RConn6 -- PS-Simulink Converter10/LConn1
